simulink model "Pollution"  (Simulink 10.0)
settings: Solver=ode45  StartTime=0.0  StopTime=5  EnableMultiTasking=on
settings Model: Creator=UX31  LastModifiedBy=unknown
settings SolverCC: ZeroCrossControl=EnableAll  ZeroCrossAlgorithm=Adaptive
settings DebuggingCC: UnderspecifiedInitializationDetection=Simplified  MergeDetectMultiDrivingBlocksExec=error
settings GRTTargetCC: GeneratePreprocessorConditionals=Disable all  CombineOutputUpdateFcns=on  GRTInterface=off
settings ConfigComp: CovExternalEMLEnable=off  CovSFcnEnable=off

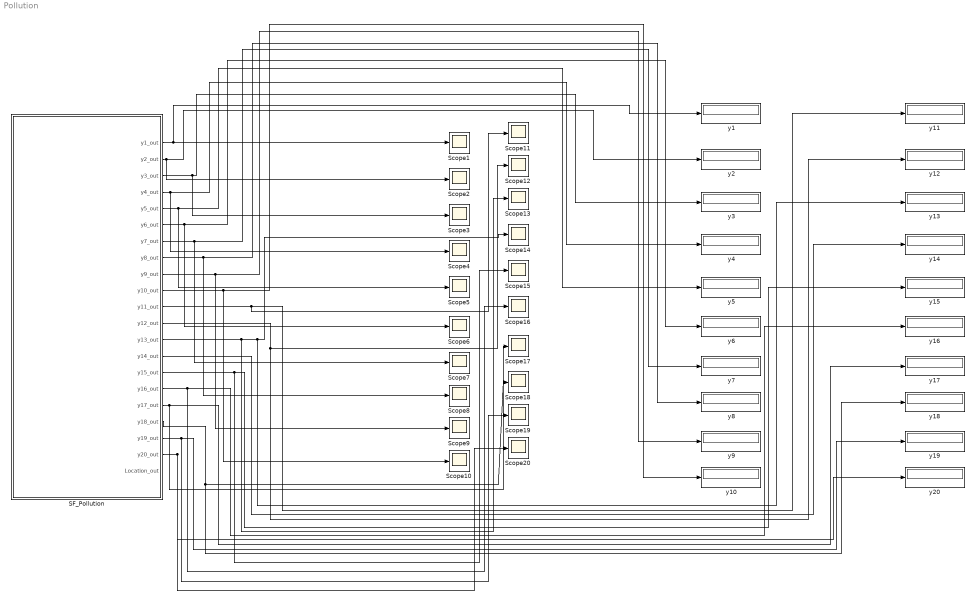
== system Pollution ==
  SF_Pollution : Stateflow chart  TreatAsAtomicUnit=on
  Scope{1..20} (20 alike) : Scope
  y{1..20} (20 alike) : Display
  wires:
  SF_Pollution/1(y1_out) -> Scope1/1, y1/1
  SF_Pollution/2(y2_out) -> Scope2/1, y2/1
  SF_Pollution/3(y3_out) -> Scope3/1, y3/1
  SF_Pollution/4(y4_out) -> Scope4/1, y4/1
  SF_Pollution/5(y5_out) -> Scope5/1, y5/1
  SF_Pollution/6(y6_out) -> Scope6/1, y6/1
  SF_Pollution/7(y7_out) -> Scope7/1, y7/1
  SF_Pollution/8(y8_out) -> Scope8/1, y8/1
  SF_Pollution/9(y9_out) -> Scope9/1, y9/1
  SF_Pollution/10(y10_out) -> Scope10/1, y10/1
  SF_Pollution/12(y12_out) -> Scope12/1, y12/1
  SF_Pollution/13(y13_out) -> Scope13/1, Scope14/1, y13/1
  SF_Pollution/14(y14_out) -> y14/1
  SF_Pollution/15(y15_out) -> Scope15/1, y15/1
  SF_Pollution/16(y16_out) -> Scope16/1, y16/1
  SF_Pollution/17(y17_out) -> Scope17/1, y17/1
  SF_Pollution/18(y18_out) -> Scope18/1, y18/1
  SF_Pollution/11(y11_out) -> Scope11/1, y11/1
  SF_Pollution/19(y19_out) -> Scope19/1, y19/1
  SF_Pollution/20(y20_out) -> Scope20/1, y20/1

== stateflow chart SF_Pollution ==
  settings: updateMethod=CONTINUOUS
  state pollution
    du:
    y1_dot=(0-k1)*y1-k10*y11*y1-k14*y1*y6-k23*y1*y4-k24*y19*y1+k2*y2*y4+k3*y5*y2+k9*y11*y2+k11*y13+k12*y10*y2+k22*y19+k25*y20;
    y2_dot=(0-k2)*y2*y4-k3*y5*y2-k9*y11*y2-k12*y10*y2+k1*y1+k21*y19;
    y3_dot=(0-k15)*y3+k1*y1+k17*y4+k19*y16+k22*y19;
    y4_dot=(0-k2)*y2*y4-k16*y4-k17*y4-k23*y1*y4+k15*y3;
    y5_dot=(0-k3)*y5*y2+2*k4*y7+k6*y7*y6+k7*y9+k13*y14+k20*y17*y6;
    y6_dot=(0-k6)*y7*y6-k8*y9*y6-k14*y1*y6-k20*y17*y6+k3*y5*y2+2*k18*y16;
    y7_dot=(0-k4)*y7-k5*y7-k6*y7*y6+k13*y14;
    y8_dot=k4*y7+k5*y7+k6*y7*y6+k7*y9;
    y9_dot=(0-k7)*y9-k8*y9*y6;
    y10_dot=(0-k12)*y10*y2+k7*y9+k9*y11*y2;
    y11_dot=(0-k9)*y11*y2-k10*y11*y1+k8*y9*y6+k11*y13;
    y12_dot=k9*y11*y2;
    y13_dot=(0-k11)*y13+k10*y11*y1;
    y14_dot=(0-k13)*y14+k12*y10*y2;
    y15_dot=k14*y1*y6;
    y16_dot=(0-k18)*y16-k19*y16+k16*y4;
    y17_dot=(0-k20)*y17*y6;
    y18_dot=k20*y17*y6;
    y19_dot=(0-k21)*y19-k22*y19-k24*y19*y1+k23*y1*y4+k25*y20;
    y20_dot=(0-k25)*y20+k24*y19*y1;
    y1_out=y1;
    y2_out=y2;
    y3_out=y3;
    y4_out=y4;
    y5_out=y5;
    y6_out=y6;
    y7_out=y7;
    y8_out=y8;
    y9_out=y9;
    y10_out=y10;
    y11_out=y11;
    y12_out=y12;
    y13_out=y13;
    y14_out=y14;
    y15_out=y15;
    y16_out=y16;
    y17_out=y17;
    y18_out=y18;
    y19_out=y19;
    y20_out=y20;
    Location_out =1;
  (default) -> pollution : {y1=0; y2=0.2;y3=0;y4=0.04;y5=0;y6=0;y7=0.1;y8=0.3;y9=0.01;y10=0;y11=0;y12=0;y13=0;y14=0;y15=0;y16=0;y17=0.007;y18=0;y19=0;y20=0}
  data: y1 local double; y1_out output double; y2 local double; y2_out output double; y3 local double; y3_out output double; y4 local double; y4_out output double; y5 local double; y5_out output double; y6 local double; y6_out output double; y7 local double; y7_out output double; y8 local double; y8_out output double; y9 local double; y9_out output double; y10 local double; y10_out output double; y11 local double; y11_out output double; y12 local double; y12_out output double; y13 local double; y13_out output double; y14 local double; y14_out output double; y15 local double; y15_out output double; y16 local double; y16_out output double; y17 local double; y17_out output double; y18 local double; y18_out output double; y19 local double; y19_out output double; y20 local double; y20_out output double; Location_out output double; k1 constant double =0.350; k2 constant double =0.266*10^2; k3 constant double =0.123*10^5; k4 constant double =0.860*10^-3; k5 constant double =0.820*10^-3; k6 constant double =0.150*10^5; k7 constant double =0.130*10^-3; k8 constant double =0.240*10^5; k9 constant double =0.165*10^5; k10 constant double =0.900*10^4; k11 constant double =0.220*10^-1; k12 constant double =0.120*10^5; k13 constant double =0.188*10; k14 constant double =0.163*10^5; k15 constant double =0.480*10^7; k16 constant double =0.350*10^-3; k17 constant double =0.175 * 10^-1; k18 constant double =0.100*10^9; k19 constant double =0.444*10^12; k20 constant double =0.124*10^4; k21 constant double =0.210*10; k22 constant double =0.578*10; k23 constant double =0.474*10^-1; k24 constant double =0.178*10^4; k25 constant double =0.312*10
  data y1 settings: updateMethod=SF_CONTINUOUS_TIME_DATA
  data y2 settings: updateMethod=SF_CONTINUOUS_TIME_DATA
  data y3 settings: updateMethod=SF_CONTINUOUS_TIME_DATA
  data y4 settings: updateMethod=SF_CONTINUOUS_TIME_DATA
  data y5 settings: updateMethod=SF_CONTINUOUS_TIME_DATA
  data y6 settings: updateMethod=SF_CONTINUOUS_TIME_DATA
  data y7 settings: updateMethod=SF_CONTINUOUS_TIME_DATA
  data y8 settings: updateMethod=SF_CONTINUOUS_TIME_DATA
  data y9 settings: updateMethod=SF_CONTINUOUS_TIME_DATA
  data y10 settings: updateMethod=SF_CONTINUOUS_TIME_DATA
  data y11 settings: updateMethod=SF_CONTINUOUS_TIME_DATA
  data y12 settings: updateMethod=SF_CONTINUOUS_TIME_DATA
  data y13 settings: updateMethod=SF_CONTINUOUS_TIME_DATA
  data y14 settings: updateMethod=SF_CONTINUOUS_TIME_DATA
  data y15 settings: updateMethod=SF_CONTINUOUS_TIME_DATA
  data y16 settings: updateMethod=SF_CONTINUOUS_TIME_DATA
  data y17 settings: updateMethod=SF_CONTINUOUS_TIME_DATA
  data y18 settings: updateMethod=SF_CONTINUOUS_TIME_DATA
  data y19 settings: updateMethod=SF_CONTINUOUS_TIME_DATA
  data y20 settings: updateMethod=SF_CONTINUOUS_TIME_DATA
